simulink model "Simulation"  (R2023b)
settings: Solver=VariableStepAuto  StartTime=0.0  StopTime=0.32  RelTol=1e-3
libraries: slpidlib x1
settings Model: Creator=Hamid Reza  LastModifiedBy=Hamid Reza

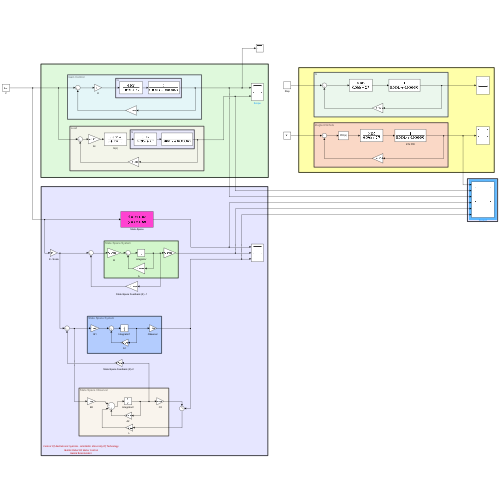
[thumbnail: Simulink's stored preview of the top-level diagram]
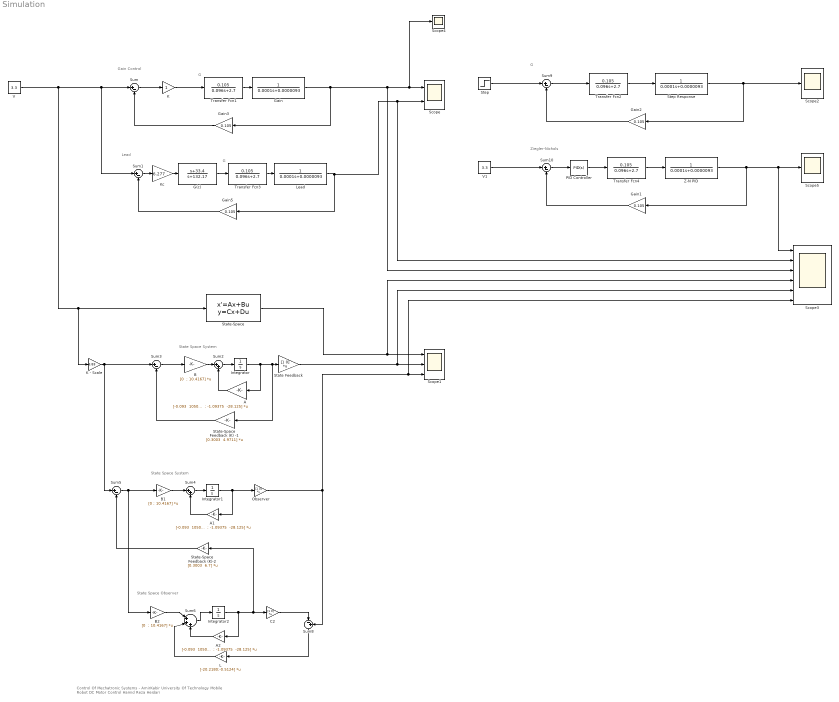
== system Simulation ==
  note: Control Of Mechatronic Systems - AmirKabir University Of Technology
      | Mobile Robot DC Motor Control
      | Hamid Reza Heidari
  note: G
  note: G
  note: Gain Control
  note: Lead
  note: State Space System
  note: State Space Observer
  note: State Space System
  note: G
  note: Ziegler-Nichols
  A : Gain  Gain="[-0.093  1050  ; -1.09375  -28.125]"  Multiplication=Matrix(K*u) (u vector)
  A1 : Gain  Gain="[-0.093  1050  ; -1.09375  -28.125]"  Multiplication=Matrix(K*u) (u vector)
  A2 : Gain  Gain="[-0.093  1050  ; -1.09375  -28.125]"  Multiplication=Matrix(K*u) (u vector)
  B : Gain  Gain="[0  ; 10.4167]"  Multiplication=Matrix(K*u) (u vector)
  B1 : Gain  Gain=[0 ; 10.4167]  Multiplication=Matrix(K*u) (u vector)
  B2 : Gain  Gain="[0  ; 10.4167]"  Multiplication=Matrix(K*u) (u vector)
  C2 : Gain  Gain=[1 0]  Multiplication=Matrix(K*u) (u vector)
  G(c) : TransferFcn  Numerator=[1 33.4]  Denominator=[1 132.17]
  Gain : TransferFcn  Denominator=[0.0001 0.0000093]
  Gain{1..3,5} (4 alike) : Gain  Gain=0.105
  Integrator : Integrator
  Integrator1 : Integrator
  Integrator2 : Integrator
  K : Gain
  K - Scale : Gain  Gain=3.83
  Kc : Gain  Gain=6.277
  L : Gain  Gain=[-20.2180;-0.5124]  Multiplication=Matrix(K*u) (u vector)
  Lead : TransferFcn  Denominator=[0.0001 0.0000093]
  "Observer " : Gain  Gain=[1 0]  Multiplication=Matrix(K*u) (u vector)
  PID Controller : slpidlib/PID Controller  Controller=PID  Form=Ideal  TimeDomain=Continuous-time  UseExternalTs=off  SampleTime=-1  IntegratorMethod=Forward Euler  FilterMethod=Forward Euler  ControllerParametersSource=internal  P=3.2571  I=0.042  UseKiTs=off  D=0.0285  N=100  UseFilter=on  TunerSelectOption=Transfer Function Based (PID Tuner App)  InitialConditionSource=internal  InitialConditionForIntegrator=0  InitialConditionForFilter=0  DifferentiatorICPrevScaledInput=0  ExternalReset=none  TrackingMode=off  Kt=1  LimitOutput=off  SatLimitsSource=internal  UpperSaturationLimit=inf  LowerSaturationLimit=-inf  LinearizeAsGain=on  AntiWindupMode=none  Kb=1  LimitIntegrator=off  UpperIntegratorSaturationLimit=inf  LowerIntegratorSaturationLimit=-inf  POutMin=[]  POutMax=[]  IOutMin=[]  IOutMax=[]  DOutMin=[]  DOutMax=[]  NOutMin=[]  NOutMax=[]  SumOutMin=[]  SumOutMax=[]  SaturationOutMin=[]  SaturationOutMax=[]  PParamMin=[]  PParamMax=[]  IParamMin=[]  IParamMax=[]  DParamMin=[]  DParamMax=[]  NParamMin=[]  NParamMax=[]  KbParamMin=[]  KbParamMax=[]  KtParamMin=[]  KtParamMax=[]  KbOutMin=[]  KbOutMax=[]  KtOutMin=[]  KtOutMax=[]  IntegratorOutMin=[]  IntegratorOutMax=[]  FilterOutMin=[]  FilterOutMax=[]  SumI1OutMin=[]  SumI1OutMax=[]  SumI2OutMin=[]  SumI2OutMax=[]  SumI3OutMin=[]  SumI3OutMax=[]  SumI4OutMin=[]  SumI4OutMax=[]  SumDOutMin=[]  SumDOutMax=[]  DifferentiatorOutMin=[]  DifferentiatorOutMax=[]  FilterDiffOutCoefMin=[]  FilterDiffOutCoefMax=[]  ReciprocalOutMin=[]  ReciprocalOutMax=[]  SumDenOutMin=[]  SumDenOutMax=[]  SumNumOutMin=[]  SumNumOutMax=[]  DivideOutMin=[]  DivideOutMax=[]  UdiffTsProdOutMin=[]  UdiffTsProdOutMax=[]  NTsProdOutMin=[]  NTsProdOutMax=[]  UintegralTsProdOutMin=[]  UintegralTsProdOutMax=[]  UngainTsProdOutMin=[]  UngainTsProdOutMax=[]  ClampingZeroOutDataTypeStr=Inherit: Inherit via back propagation  ClampingZeroOutMin=[]  ClampingZeroOutMax=[]  FilterDenConstantOutDataTypeStr=Inherit: Inherit via back propagation  FilterDenConstantOutMin=[]  FilterDenConstantOutMax=[]  PCopyOutDataTypeStr=Inherit: Inherit via back propagation  PCopyOutMin=[]  PCopyOutMax=[]  NCopyOutDataTypeStr=Inherit: Inherit via back propagation  NCopyOutMin=[]  NCopyOutMax=[]  IntegratorContinuousStateAttributes=''  IntegratorStateMustResolveToSignalObject=off  IntegratorRTWStateStorageClass=Auto  FilterContinuousStateAttributes=''  FilterStateMustResolveToSignalObject=off  FilterRTWStateStorageClass=Auto  ParallelPVariant=Passthrough  IdealPVariant=InternalParameters  IVariant=InternalParameters  DVariant=InternalParameters  IntegratorVariant=Continuous  SatVariant=Disabled  AWVariant=Passthrough  PCopyVariant=Disabled  TRVariant=Disabled  FdbkBlocksVariant=Forward  IdealPFdbkVariant=Disabled  SatFdbkVariant=Disabled  DerivativeFilterVariant=ContFilter  NVariant=InternalParameters  NCopyVariant=Disabled  FilterICVariant=InternalICsFilter  IntegratorICVariant=InternalICs  ExternalResetVariant=Disabled  TRSumVariant=Passthrough  SumFdbkVariant=Disabled  SumVariant=Sum_PID  TsampFilterVariant=InternalTs  TsampNgainVariant=Passthrough  TsampIntegralVariant=Disabled_SignalSpec  ExternalSaturationOutDataTypeStr=Inherit: Same as second input
  Scope : Scope  NumInputPorts=2
  Scope1 : Scope  NumInputPorts=3
  Scope2 : Scope
  Scope3 : Scope  NumInputPorts=6
  Scope4 : Scope
  Scope5 : Scope
  State Feedback : Gain  Gain=[1 0]  Multiplication=Matrix(K*u) (u vector)
  State-Space : StateSpace  A="[-0.093 1050 ; -1.09375  -28.125]"  B=[0 ; 10.4167]  C=[1 0]  D=0  InitialCondition=0
  State-Space Feedback (K) -1 : Gain  Gain="[0.3003  4.9711]"  Multiplication=Matrix(K*u) (u vector)
  State-Space Feedback (K)-2 : Gain  Gain="[0.3003  6.7]"  Multiplication=Matrix(K*u) (u vector)
  Step : Step  Time=0  SampleTime=0
  Step Response : TransferFcn  Denominator=[0.0001 0.0000093]
  Sum{,1,3,5,9..10} (6 alike) : Sum  Inputs=|+-
  Sum2 : Sum  Inputs=|++
  Sum4 : Sum  Inputs=|++
  Sum6 : Sum  Inputs=|+++
  Sum8 : Sum  Inputs=|-+
  Transfer Fcn{1..4} (4 alike) : TransferFcn  Numerator=[0.105]  Denominator=[0.096 2.7]
  V : Constant  Value=3.3
  V1 : Constant  Value=3.3
  Z-N PID : TransferFcn  Denominator=[0.0001 0.0000093]
  wires:
  Transfer Fcn1/1 -> Gain/1
  Gain/1 -> Gain3/1, Scope3/3, Scope4/1, Scope/1
  Gain3/1 -> Sum/2
  K/1 -> Transfer Fcn1/1
  Sum/1 -> K/1
  Sum1/1 -> Kc/1
  Gain5/1 -> Sum1/2
  Lead/1 -> Scope/2, Scope3/2, Gain5/1
  Transfer Fcn3/1 -> Lead/1
  Kc/1 -> G(c)/1
  G(c)/1 -> Transfer Fcn3/1
  Sum6/1 -> Integrator2/1
  V/1 -> State-Space/1, K - Scale/1, Sum1/1, Sum/1
  A2/1 -> Sum6/3
  Sum8/1 -> L/1
  L/1 -> Sum6/2
  B1/1 -> Sum4/1
  A1/1 -> Sum4/2
  C2/1 -> Sum8/1
  Integrator1/1 -> "Observer "/1, A1/1
  State-Space Feedback (K)-2/1 -> Sum5/2
  Sum4/1 -> Integrator1/1
  Integrator2/1 -> A2/1, State-Space Feedback (K)-2/1, C2/1
  Sum5/1 -> B1/1, B2/1
  B/1 -> Sum2/1
  State-Space/1 -> Scope3/4, Scope1/1
  Integrator/1 -> A/1, State-Space Feedback (K) -1/1, State Feedback/1
  State Feedback/1 -> Scope3/5, Scope1/2
  "Observer "/1 -> Scope3/6, Scope1/3, Sum8/2
  A/1 -> Sum2/2
  B2/1 -> Sum6/1
  Sum2/1 -> Integrator/1
  State-Space Feedback (K) -1/1 -> Sum3/2
  Sum9/1 -> Transfer Fcn2/1
  Gain2/1 -> Sum9/2
  Step Response/1 -> Gain2/1, Scope2/1
  Transfer Fcn2/1 -> Step Response/1
  Sum3/1 -> B/1
  K - Scale/1 -> Sum3/1, Sum5/1
  Transfer Fcn4/1 -> Z-N PID/1
  Gain1/1 -> Sum10/2
  V1/1 -> Sum10/1
  Sum10/1 -> PID Controller/1
  PID Controller/1 -> Transfer Fcn4/1
  Z-N PID/1 -> Scope5/1, Scope3/1, Gain1/1
  Step/1 -> Sum9/1
